simulink model "Optitrack_test"  (R2023a)
settings: Solver=ode8  StartTime=0.0  StopTime=180  FixedStep=0.1  RelTol=1e-3
libraries: ros2lib x2
settings Model: Creator=vinny-desktop-win10  LastModifiedBy=vinny-desktop-win10

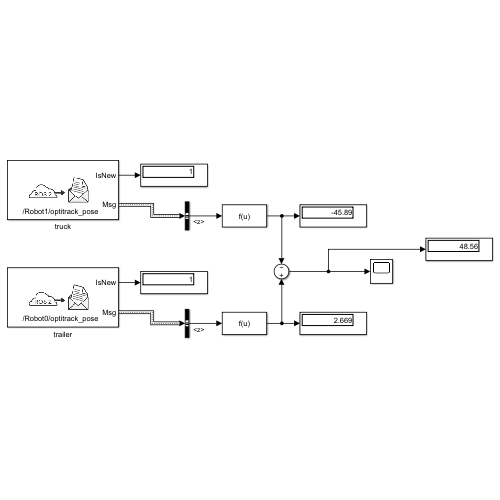
[thumbnail: Simulink's stored preview of the top-level diagram]
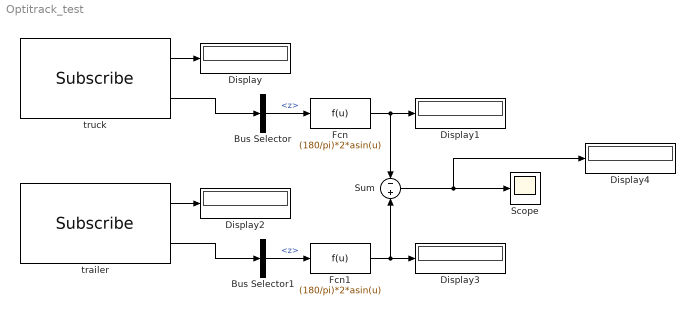
== system Optitrack_test ==
  Bus Selector : BusSelector  OutputSignals=pose.orientation.z
  Bus Selector1 : BusSelector  OutputSignals=pose.orientation.z
  Display{,1..4} (5 alike) : Display
  Fcn : Fcn  Expr=(180/pi)*2*asin(u)
  Fcn1 : Fcn  Expr=(180/pi)*2*asin(u)
  Scope : Scope
  Sum : Sum  Inputs=-|+
  trailer : ros2lib/Subscribe  topicSource=Select from ROS network  topic=/Robot0/optitrack_pose  messageType=geometry_msgs/PoseStamped  sampleTime=-1  QOSHistory=Keep last  QOSDepth=1  QOSReliability=Reliable  QOSDurability=Volatile
  truck : ros2lib/Subscribe  topicSource=Select from ROS network  topic=/Robot1/optitrack_pose  messageType=geometry_msgs/PoseStamped  sampleTime=-1  QOSHistory=Keep last  QOSDepth=1  QOSReliability=Reliable  QOSDurability=Volatile
  wires:
  truck/1 -> Display/1
  truck/2 -> Bus Selector/1
  Bus Selector/1 -> Fcn/1  "<z>"
  Fcn/1 -> Display1/1, Sum/1
  Fcn1/1 -> Display3/1, Sum/2
  trailer/2 -> Bus Selector1/1
  trailer/1 -> Display2/1
  Bus Selector1/1 -> Fcn1/1  "<z>"
  Sum/1 -> Display4/1, Scope/1
